simulink model "voltage_integrator"  (R2013a)
settings: Solver=ode45  StartTime=0.0  StopTime=10.0  FixedStep=1/FPGA_Output_Freq  MaxStep=1/FPGA_Output_Freq  RelTol=1e-5
undefined symbols (not defined in the file or in its folder): C_int, R_mes_high, R_mes_low, R_neg, R_pos, V_int_max, V_int_min
settings Model: ParamWorkspaceSource=ReferencedWorkspace  TunableVars=C_int,R_mes_high,R_mes_low,R_neg,R_pos,V_int_max,V_int_min  TunableVarsStorageClass=Auto,Auto,Auto,Auto,Auto,Auto,Auto  TunableVarsTypeQualifier=,,,,,,  Creator=Lukas  LastModifiedBy=Steinert
settings OptimizationCC: InlineParams=on  ExpressionDepthLimit=2147483647
settings ModelReferenceCC: ModelReferenceMinAlgLoopOccurrences=on

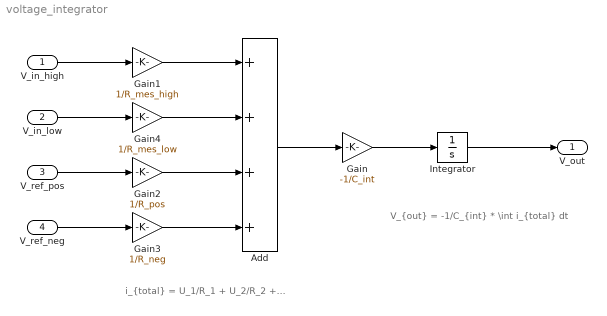
== system voltage_integrator ==
  note: i_{total} = U_1/R_1 + U_2/R_2 +...
  note: V_{out} = -1/C_{int} * \int i_{total} dt
  V_in_high : Inport
  V_in_low : Inport  Port=2
  V_ref_pos : Inport  Port=3
  V_ref_neg : Inport  Port=4
  Add : Sum  Inputs=++++
  Gain : Gain  Gain=-1/C_int
  Gain1 : Gain  Gain=1/R_mes_high
  Gain2 : Gain  Gain=1/R_pos
  Gain3 : Gain  Gain=1/R_neg
  Gain4 : Gain  Gain=1/R_mes_low
  Integrator : Integrator  LimitOutput=on  UpperSaturationLimit=V_int_max  LowerSaturationLimit=V_int_min
  V_out : Outport
  wires:
  Gain1/1 -> Add/1
  Gain4/1 -> Add/2
  Gain2/1 -> Add/3
  Gain3/1 -> Add/4
  Add/1 -> Gain/1
  Gain/1 -> Integrator/1
  V_in_high/1 -> Gain1/1
  V_in_low/1 -> Gain4/1
  V_ref_pos/1 -> Gain2/1
  V_ref_neg/1 -> Gain3/1
  Integrator/1 -> V_out/1
